simulink model "KaszkadMotorSzabalyozo"  (R2020b)
settings: Solver=VariableStepAuto  StartTime=0.0  StopTime=10.0  RelTol=1e-3
values from neighbouring files (symbols this model uses):
  Ai = c2/(R+Ki)    (= 0.00267882187938)    [kaszkadSzabalyozo.m]
  c1 = 1/26.6    (= 0.0375939849624)    [kaszkadSzabalyozo.m]
  c2 = 0.0382    [kaszkadSzabalyozo.m]
  Fv = 0.001795    [kaszkadSzabalyozo.m]
  J = 0.0001    [kaszkadSzabalyozo.m]
  Ki = R    (= 7.13)    [kaszkadSzabalyozo.m]
  Kp = (J*omega_n^2)/Ai    (= 3.73298429319)    [kaszkadSzabalyozo.m]
  Kv = ((2*csillapitas*omega_n*J-Fv)/Ai)-c1    (= 0.113591878912)    [kaszkadSzabalyozo.m]
  L = 1.05    [kaszkadSzabalyozo.m]
  R = 7.13    [kaszkadSzabalyozo.m]
  Tau_ext = 0.01    [kaszkadSzabalyozo.m]
settings Model: Creator=Legion1  LastModifiedBy=Legion1

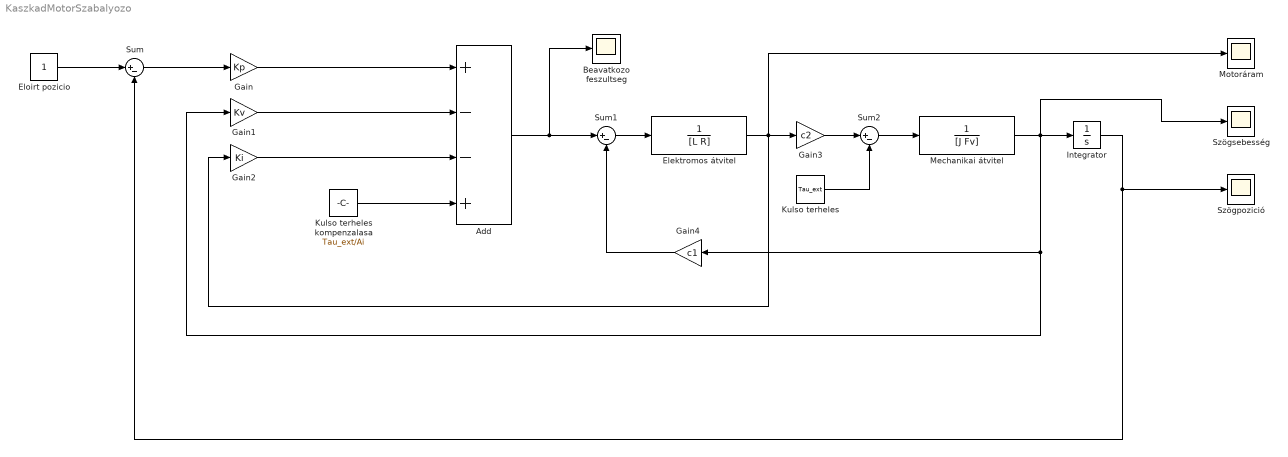
== system KaszkadMotorSzabalyozo ==
  Add : Sum  Inputs=+--+
  Beavatkozo feszultseg : Scope
  Elektromos átvitel : TransferFcn  Denominator=[L R]
  Eloirt pozicio : Constant
  Gain : Gain  Gain=Kp
  Gain1 : Gain  Gain=Kv
  Gain2 : Gain  Gain=Ki
  Gain3 : Gain  Gain=c2
  Gain4 : Gain  Gain=c1
  Integrator : Integrator
  Kulso terheles : Constant  Value=Tau_ext
  Kulso terheles kompenzalasa : Constant  Value=Tau_ext/Ai
  Mechanikai átvitel : TransferFcn  Denominator=[J Fv]
  Motoráram : Scope
  Sum : Sum  Inputs=|+-
  Sum1 : Sum  Inputs=|+-
  Sum2 : Sum  Inputs=|+-
  Szögpozició : Scope
  Szögsebesség : Scope
  wires:
  Eloirt pozicio/1 -> Sum/1
  Gain/1 -> Add/1
  Gain1/1 -> Add/2
  Gain2/1 -> Add/3
  Kulso terheles kompenzalasa/1 -> Add/4
  Sum/1 -> Gain/1
  Add/1 -> Beavatkozo feszultseg/1, Sum1/1
  Sum1/1 -> Elektromos átvitel/1
  Elektromos átvitel/1 -> Motoráram/1, Gain2/1, Gain3/1
  Sum2/1 -> Mechanikai átvitel/1
  Gain3/1 -> Sum2/1
  Kulso terheles/1 -> Sum2/2
  Mechanikai átvitel/1 -> Szögsebesség/1, Gain4/1, Gain1/1, Integrator/1
  Integrator/1 -> Szögpozició/1, Sum/2
  Gain4/1 -> Sum1/2
